simulink model "requirementtable_3k04project"  (R2022b)
settings: Solver=FixedStepAuto  StartTime=0.0  StopTime=10.0  FixedStep=1e-3  RelTol=1e-3  EnableMultiTasking=on
settings Model: ExtModeTrigDuration=5  Creator=16479  LastModifiedBy=jathe
settings SolverCC: AlgebraicLoopSolver=TrustRegion
settings OptimizationCC: EnhancedBackFolding=on  PassReuseOutputArgsAs=Individual arguments  ZeroExternalMemoryAtStartup=off  ZeroInternalMemoryAtStartup=off  MaxStackSize=64  OptimizeBlockOrder=speed  DifferentSizesBufferReuse=on  OptimizationCustomize=off  EfficientTunableParamExpr=on
settings DebuggingCC: ParameterTunabilityLossMsg=error  UnconnectedInputMsg=warning  UnconnectedOutputMsg=warning  UnconnectedLineMsg=warning  SFMachineParentedDataDiag=warning
settings HardwareCC: ProdBitPerPointer=32  ProdBitPerSizeT=32  ProdBitPerPtrDiffT=32  ProdLargestAtomicInteger=Long  ProdLargestAtomicFloat=Double  ProdWordSize=32  ProdHWDeviceType=ARM Compatible->ARM Cortex
settings ModelReferenceCC: EnableRefExpFcnMdlSchedulingChecks=on
settings SFSimCC: MATLABDynamicMemAlloc=off
settings RTWCC: Description=Embedded Coder  SystemTargetFile=ert.tlc  HardwareBoard=NXP FRDM-K64F  TLCOptions="-aInlineSetEventsForThisBaseRateFcn=TLC_FALSE -aSuppressMultiTaskScheduler=TLC_FALSE  -aRateBasedStepFcn=0"  TemplateMakefile=ert_default_tmf  Toolchain=GNU Tools for ARM Embedded Processors  DLArmComputeVersion=19.05
settings CodeAppCC: ForceParamTrailComments=on  IgnoreCustomStorageClasses=off  OperatorAnnotations=on  SimulinkDataObjDesc=on  SFDataObjDesc=on  InsertBlockDesc=on
settings ERTTargetCC: ExtModeTransport=4  ExtModeMexFile=sendToCommService

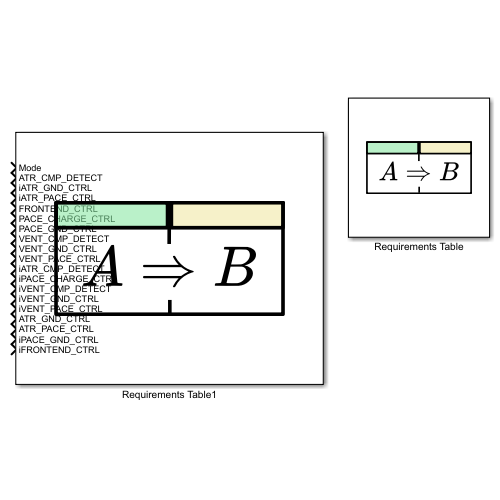
[thumbnail: Simulink's stored preview of the top-level diagram]
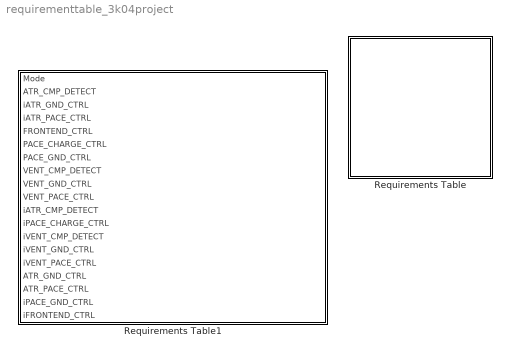
== system requirementtable_3k04project ==
  Requirements Table : Requirements Table  TreatAsAtomicUnit=on
  Requirements Table1 : Requirements Table  TreatAsAtomicUnit=on

== stateflow chart requirementtable_3k04project/Requirements Table1 ==
  (default) -> (junction 1073747097)
  (junction 1073747097) -> (junction 1073747098) : {
      | % SF_REQ_REV_07
      | }
  (junction 1073747098) -> (junction 1073747136) : {
      | % HEADER_ASSIGNMENTS
      |
      | }
  (junction 1073747136) -> (junction 1073747138) : {
      | % START_A_52
      | }
  (junction 1073747138) -> (junction 1073747140) : {
      | }
  (junction 1073747140) -> (junction 1073747142)
  (junction 1073747142) -> (junction 1073747144) [order 1] : [(iPACE_GND_CTRL==true)]
  (junction 1073747142) -> (junction 1073747150) [order 2]
  (junction 1073747144) -> (junction 1073747146)
  (junction 1073747146) -> (junction 1073747148) : {
      | }
  (junction 1073747148) -> (junction 1073747150)
  (junction 1073747150) -> (junction 1073747152)
  (junction 1073747152) -> (junction 1073747154) : {
      | % END_A_52
      | }
  (junction 1073747154) -> (junction 1073747156) : {
      | % START_R_1
      | }
  (junction 1073747156) -> (junction 1073747158) : {
      | }
  (junction 1073747158) -> (junction 1073747160)
  (junction 1073747160) -> (junction 1073747162) [order 1] : [(iPACE_CHARGE_CTRL==false) && (iVENT_PACE_CTRL==true) && (iVENT_GND_CTRL==false) && (Mode==1)]
  (junction 1073747160) -> (junction 1073747168) [order 2]
  (junction 1073747162) -> (junction 1073747164) : {
      | reqtable_postcondition((PACE_CHARGE_CTRL==true) && (VENT_GND_CTRL==true) && (VENT_PACE_CTRL==false), 'R:1');
      |
      |
      | }
  (junction 1073747164) -> (junction 1073747166) : {
      | }
  (junction 1073747166) -> (junction 1073747168)
  (junction 1073747168) -> (junction 1073747170)
  (junction 1073747170) -> (junction 1073747172) : {
      | % END_R_1
      | }
  (junction 1073747172) -> (junction 1073747174) : {
      | % START_R_16
      | }
  (junction 1073747174) -> (junction 1073747176) : {
      | }
  (junction 1073747176) -> (junction 1073747178)
  (junction 1073747178) -> (junction 1073747180) [order 1] : [(iPACE_CHARGE_CTRL==false) && (iATR_GND_CTRL==false) && (iATR_PACE_CTRL==true) && (Mode==2)]
  (junction 1073747178) -> (junction 1073747186) [order 2]
  (junction 1073747180) -> (junction 1073747182) : {
      | reqtable_postcondition((PACE_CHARGE_CTRL==true) && (ATR_GND_CTRL==true) && (ATR_PACE_CTRL==false), 'R:2');
      |
      |
      | }
  (junction 1073747182) -> (junction 1073747184) : {
      | }
  (junction 1073747184) -> (junction 1073747186)
  (junction 1073747186) -> (junction 1073747188)
  (junction 1073747188) -> (junction 1073747190) : {
      | % END_R_16
      | }
  (junction 1073747190) -> (junction 1073747192) : {
      | % START_R_13
      | }
  (junction 1073747192) -> (junction 1073747194) : {
      | }
  (junction 1073747194) -> (junction 1073747196)
  (junction 1073747196) -> (junction 1073747198) [order 1] : [(iPACE_CHARGE_CTRL==true) && (iVENT_GND_CTRL==true) && (iVENT_PACE_CTRL==false) && (Mode~=3)]
  (junction 1073747196) -> (junction 1073747204) [order 2]
  (junction 1073747198) -> (junction 1073747200) : {
      | reqtable_postcondition((PACE_CHARGE_CTRL==false) && (VENT_GND_CTRL==false) && (VENT_PACE_CTRL==true), 'R:3');
      |
      |
      | }
  (junction 1073747200) -> (junction 1073747202) : {
      | }
  (junction 1073747202) -> (junction 1073747204)
  (junction 1073747204) -> (junction 1073747206)
  (junction 1073747206) -> (junction 1073747208) : {
      | % END_R_13
      | }
  (junction 1073747208) -> (junction 1073747210) : {
      | % START_R_19
      | }
  (junction 1073747210) -> (junction 1073747212) : {
      | }
  (junction 1073747212) -> (junction 1073747214)
  (junction 1073747214) -> (junction 1073747216) [order 1] : [(iPACE_CHARGE_CTRL==true) && (iATR_GND_CTRL==true) && (iATR_PACE_CTRL==false) && (Mode~=4)]
  (junction 1073747214) -> (junction 1073747222) [order 2]
  (junction 1073747216) -> (junction 1073747218) : {
      | reqtable_postcondition((PACE_CHARGE_CTRL==false) && (ATR_GND_CTRL==false) && (ATR_PACE_CTRL==true), 'R:4');
      |
      |
      | }
  (junction 1073747218) -> (junction 1073747220) : {
      | }
  (junction 1073747220) -> (junction 1073747222)
  (junction 1073747222) -> (junction 1073747224)
  (junction 1073747224) -> (junction 1073747226) : {
      | % END_R_19
      | }
  (junction 1073747226) -> (junction 1073747228) : {
      | % START_R_22
      | }
  (junction 1073747228) -> (junction 1073747230) : {
      | }
  (junction 1073747230) -> (junction 1073747232)
  (junction 1073747232) -> (junction 1073747234) [order 1] : [(iPACE_CHARGE_CTRL==true) && (iVENT_GND_CTRL==true) && (iVENT_PACE_CTRL==false) && (Mode==3)]
  (junction 1073747232) -> (junction 1073747240) [order 2]
  (junction 1073747234) -> (junction 1073747236) : {
      | reqtable_postcondition((FRONTEND_CTRL==true), 'R:5');
      |
      |
      | }
  (junction 1073747236) -> (junction 1073747238) : {
      | }
  (junction 1073747238) -> (junction 1073747240)
  (junction 1073747240) -> (junction 1073747242)
  (junction 1073747242) -> (junction 1073747244) : {
      | % END_R_22
      | }
  (junction 1073747244) -> (junction 1073747246) : {
      | % START_R_34
      | }
  (junction 1073747246) -> (junction 1073747248) : {
      | }
  (junction 1073747248) -> (junction 1073747250)
  (junction 1073747250) -> (junction 1073747252) [order 1] : [(iPACE_CHARGE_CTRL==true) && (iATR_GND_CTRL==true) && (iATR_PACE_CTRL==false) && (Mode==4)]
  (junction 1073747250) -> (junction 1073747258) [order 2]
  (junction 1073747252) -> (junction 1073747254) : {
      | reqtable_postcondition((FRONTEND_CTRL==true), 'R:6');
      |
      |
      | }
  (junction 1073747254) -> (junction 1073747256) : {
      | }
  (junction 1073747256) -> (junction 1073747258)
  (junction 1073747258) -> (junction 1073747260)
  (junction 1073747260) -> (junction 1073747262) : {
      | % END_R_34
      | }
  (junction 1073747262) -> (junction 1073747264) : {
      | % START_R_61
      | }
  (junction 1073747264) -> (junction 1073747266) : {
      | }
  (junction 1073747266) -> (junction 1073747268)
  (junction 1073747268) -> (junction 1073747270) [order 1] : [(iVENT_CMP_DETECT==true) && (Mode==3)]
  (junction 1073747268) -> (junction 1073747276) [order 2]
  (junction 1073747270) -> (junction 1073747272) : {
      |
      |
      | }
  (junction 1073747272) -> (junction 1073747274) : {
      | }
  (junction 1073747274) -> (junction 1073747276)
  (junction 1073747276) -> (junction 1073747278)
  (junction 1073747278) -> (junction 1073747280) : {
      | % END_R_61
      | }
  (junction 1073747280) -> (junction 1073747282) : {
      | % START_R_64
      | }
  (junction 1073747282) -> (junction 1073747284) : {
      | }
  (junction 1073747284) -> (junction 1073747286)
  (junction 1073747286) -> (junction 1073747288) [order 1] : [(iATR_CMP_DETECT==true) && (Mode==4)]
  (junction 1073747286) -> (junction 1073747294) [order 2]
  (junction 1073747288) -> (junction 1073747290) : {
      |
      |
      | }
  (junction 1073747290) -> (junction 1073747292) : {
      | }
  (junction 1073747292) -> (junction 1073747294)
  (junction 1073747294) -> (junction 1073747296)
  (junction 1073747296) -> (junction 1073747298) : {
      | % END_R_64
      | }
  data: Mode input; ATR_CMP_DETECT input; iATR_GND_CTRL input; iATR_PACE_CTRL input; FRONTEND_CTRL input; PACE_CHARGE_CTRL input; PACE_GND_CTRL input; VENT_CMP_DETECT input; VENT_GND_CTRL input; VENT_PACE_CTRL input; iATR_CMP_DETECT input; iPACE_CHARGE_CTRL input; iVENT_CMP_DETECT input; iVENT_GND_CTRL input; iVENT_PACE_CTRL input; ATR_GND_CTRL input; ATR_PACE_CTRL input; iPACE_GND_CTRL input; iFRONTEND_CTRL input

== stateflow chart requirementtable_3k04project/Requirements Table ==
  (default) -> (junction 1073747097)
  (junction 1073747097) -> (junction 1073747098) : {
      | % SF_REQ_REV_07
      | }
  (junction 1073747098) -> (junction 1073747136) : {
      | % HEADER_ASSIGNMENTS
      |
      | }
  (junction 1073747136) -> (junction 1073747138) : {
      | % START_A_52
      | }
  (junction 1073747138) -> (junction 1073747140) : {
      | }
  (junction 1073747140) -> (junction 1073747142)
  (junction 1073747142) -> (junction 1073747144) [order 1] : [(PACE_GND_CTRL==true)]
  (junction 1073747142) -> (junction 1073747150) [order 2]
  (junction 1073747144) -> (junction 1073747146)
  (junction 1073747146) -> (junction 1073747148) : {
      | }
  (junction 1073747148) -> (junction 1073747150)
  (junction 1073747150) -> (junction 1073747152)
  (junction 1073747152) -> (junction 1073747154) : {
      | % END_A_52
      | }
  (junction 1073747154) -> (junction 1073747156) : {
      | % START_R_1
      | }
  (junction 1073747156) -> (junction 1073747158) : {
      | }
  (junction 1073747158) -> (junction 1073747160)
  (junction 1073747160) -> (junction 1073747162) [order 1] : [(PACE_CHARGE_CTRL==false) && (VENT_PACE_CTRL==true) && (VENT_GND_CTRL==false) && (Mode==VOO)]
  (junction 1073747160) -> (junction 1073747168) [order 2]
  (junction 1073747162) -> (junction 1073747164) : {
      | reqtable_postcondition((PACE_CHARGE_CTRL==true) && (VENT_GND_CTRL==true) && (VENT_PACE_CTRL==false), 'R:1');
      |
      |
      | }
  (junction 1073747164) -> (junction 1073747166) : {
      | }
  (junction 1073747166) -> (junction 1073747168)
  (junction 1073747168) -> (junction 1073747170)
  (junction 1073747170) -> (junction 1073747172) : {
      | % END_R_1
      | }
  (junction 1073747172) -> (junction 1073747174) : {
      | % START_R_16
      | }
  (junction 1073747174) -> (junction 1073747176) : {
      | }
  (junction 1073747176) -> (junction 1073747178)
  (junction 1073747178) -> (junction 1073747180) [order 1] : [(PACE_CHARGE_CTRL==false) && (ATR_GND_CTRL==false) && (ATR_PACE_CTRL==true) && (Mode==AOO)]
  (junction 1073747178) -> (junction 1073747186) [order 2]
  (junction 1073747180) -> (junction 1073747182) : {
      | reqtable_postcondition((PACE_CHARGE_CTRL==true) && (ATR_GND_CTRL==true) && (ATR_PACE_CTRL==false), 'R:2');
      |
      |
      | }
  (junction 1073747182) -> (junction 1073747184) : {
      | }
  (junction 1073747184) -> (junction 1073747186)
  (junction 1073747186) -> (junction 1073747188)
  (junction 1073747188) -> (junction 1073747190) : {
      | % END_R_16
      | }
  (junction 1073747190) -> (junction 1073747192) : {
      | % START_R_13
      | }
  (junction 1073747192) -> (junction 1073747194) : {
      | }
  (junction 1073747194) -> (junction 1073747196)
  (junction 1073747196) -> (junction 1073747198) [order 1] : [(PACE_CHARGE_CTRL==true) && (VENT_GND_CTRL==true) && (VENT_PACE_CTRL==false) && (Mode~=VVI)]
  (junction 1073747196) -> (junction 1073747204) [order 2]
  (junction 1073747198) -> (junction 1073747200) : {
      | reqtable_postcondition((PACE_CHARGE_CTRL==false) && (VENT_GND_CTRL==false) && (VENT_PACE_CTRL==true), 'R:3');
      |
      |
      | }
  (junction 1073747200) -> (junction 1073747202) : {
      | }
  (junction 1073747202) -> (junction 1073747204)
  (junction 1073747204) -> (junction 1073747206)
  (junction 1073747206) -> (junction 1073747208) : {
      | % END_R_13
      | }
  (junction 1073747208) -> (junction 1073747210) : {
      | % START_R_19
      | }
  (junction 1073747210) -> (junction 1073747212) : {
      | }
  (junction 1073747212) -> (junction 1073747214)
  (junction 1073747214) -> (junction 1073747216) [order 1] : [(PACE_CHARGE_CTRL==true) && (ATR_GND_CTRL==true) && (ATR_PACE_CTRL==false) && (Mode~=AAI)]
  (junction 1073747214) -> (junction 1073747222) [order 2]
  (junction 1073747216) -> (junction 1073747218) : {
      | reqtable_postcondition((PACE_CHARGE_CTRL==false) && (ATR_GND_CTRL==false) && (ATR_PACE_CTRL==true), 'R:4');
      |
      |
      | }
  (junction 1073747218) -> (junction 1073747220) : {
      | }
  (junction 1073747220) -> (junction 1073747222)
  (junction 1073747222) -> (junction 1073747224)
  (junction 1073747224) -> (junction 1073747226) : {
      | % END_R_19
      | }
  (junction 1073747226) -> (junction 1073747228) : {
      | % START_R_22
      | }
  (junction 1073747228) -> (junction 1073747230) : {
      | }
  (junction 1073747230) -> (junction 1073747232)
  (junction 1073747232) -> (junction 1073747234) [order 1] : [(PACE_CHARGE_CTRL==true) && (VENT_GND_CTRL==true) && (VENT_PACE_CTRL==false) && (Mode==VVI)]
  (junction 1073747232) -> (junction 1073747240) [order 2]
  (junction 1073747234) -> (junction 1073747236) : {
      | reqtable_postcondition((FRONTEND_CTRL==true), 'R:5');
      |
      |
      | }
  (junction 1073747236) -> (junction 1073747238) : {
      | }
  (junction 1073747238) -> (junction 1073747240)
  (junction 1073747240) -> (junction 1073747242)
  (junction 1073747242) -> (junction 1073747244) : {
      | % END_R_22
      | }
  (junction 1073747244) -> (junction 1073747246) : {
      | % START_R_34
      | }
  (junction 1073747246) -> (junction 1073747248) : {
      | }
  (junction 1073747248) -> (junction 1073747250)
  (junction 1073747250) -> (junction 1073747252) [order 1] : [(PACE_CHARGE_CTRL==true) && (ATR_GND_CTRL==true) && (ATR_PACE_CTRL==false) && (Mode==AAI)]
  (junction 1073747250) -> (junction 1073747258) [order 2]
  (junction 1073747252) -> (junction 1073747254) : {
      | reqtable_postcondition((FRONTEND_CTRL==true), 'R:6');
      |
      |
      | }
  (junction 1073747254) -> (junction 1073747256) : {
      | }
  (junction 1073747256) -> (junction 1073747258)
  (junction 1073747258) -> (junction 1073747260)
  (junction 1073747260) -> (junction 1073747262) : {
      | % END_R_34
      | }
  (junction 1073747262) -> (junction 1073747264) : {
      | % START_R_61
      | }
  (junction 1073747264) -> (junction 1073747266) : {
      | }
  (junction 1073747266) -> (junction 1073747268)
  (junction 1073747268) -> (junction 1073747270) [order 1] : [(VENT_CMP_DETECT==true) && (Mode==VVI)]
  (junction 1073747268) -> (junction 1073747276) [order 2]
  (junction 1073747270) -> (junction 1073747272) : {
      |
      |
      | }
  (junction 1073747272) -> (junction 1073747274) : {
      | }
  (junction 1073747274) -> (junction 1073747276)
  (junction 1073747276) -> (junction 1073747278)
  (junction 1073747278) -> (junction 1073747280) : {
      | % END_R_61
      | }
  (junction 1073747280) -> (junction 1073747282) : {
      | % START_R_64
      | }
  (junction 1073747282) -> (junction 1073747284) : {
      | }
  (junction 1073747284) -> (junction 1073747286)
  (junction 1073747286) -> (junction 1073747288) [order 1] : [(ATR_CMP_DETECT==true) && (Mode==AAI)]
  (junction 1073747286) -> (junction 1073747294) [order 2]
  (junction 1073747288) -> (junction 1073747290) : {
      |
      |
      | }
  (junction 1073747290) -> (junction 1073747292) : {
      | }
  (junction 1073747292) -> (junction 1073747294)
  (junction 1073747294) -> (junction 1073747296)
  (junction 1073747296) -> (junction 1073747298) : {
      | % END_R_64
      | }
